simulink model "PLL_blocks"  (R2014a)
settings: Solver=ode45  StartTime=0.0  StopTime=10.0  RelTol=1e-3
libraries: simulink x12
settings Model: Creator=Tony  LastModifiedBy=Tony

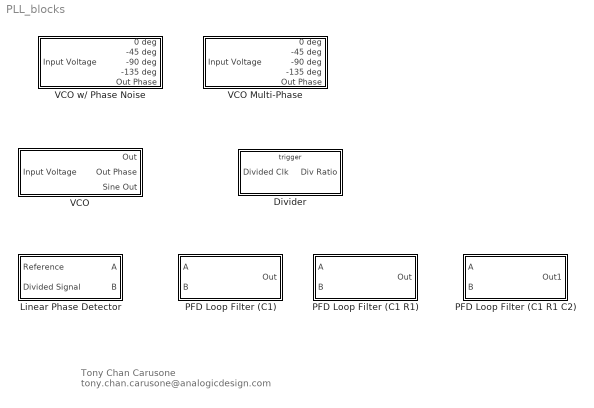
== system PLL_blocks ==
  note: Tony Chan Carusone
      | tony.chan.carusone@analogicdesign.com
  Divider : Subsystem
  Linear Phase Detector : Subsystem
  PFD Loop Filter (C1 R1 C2) : Subsystem  mask{Iu=25e-6, Id=25e-6, R1=6400, C1=16e-12, C2=1.6e-12}
      mask prompts: Iu "Loop Filter Pull Up Current (Iu)"; Id "Loop Filter Pull Down Current (Id)"
  PFD Loop Filter (C1 R1) : Subsystem  mask{Iu=25e-6, Id=25e-6, R1=8400, C1=16e-12}
      mask prompts: Iu "Loop Filter Pull Up Current (Iu)"; Id "Loop Filter Pull Down Current (Id)"
  PFD Loop Filter (C1) : Subsystem  mask{Iu=25e-6, Id=25e-6, C1=16e-12}
      mask prompts: Iu "Loop Filter Pull Up Current (Iu)"; Id "Loop Filter Pull Down Current (Id)"
  VCO : Subsystem  mask{Kvco=1e9*2*pi, Ac=1, fo=1000e6}
      mask prompts: fo "Default Frequency (fo)"
  VCO Multi-Phase : Subsystem  mask{Kvco=1e9*2*pi, fo=1000e6}
      mask prompts: fo "Default Frequency (fo)"
  VCO w/ Phase Noise : Subsystem  mask{Kvco=1e9*2*pi, fo=1000e6, h0=3e-15, N1=0}
      mask prompts: Kvco "Kvco [rad/s/V]"; fo "Nominal Frequency (fo) [Hz]"; h0 "White phase noise spectal density (rad^2/Hz)"; N1 "Low frequency phase noise (Hz^2*rad^2/Hz)"

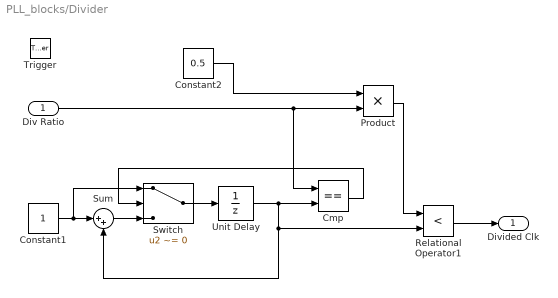
== system PLL_blocks/Divider ==
  Div Ratio : Inport
  Trigger : TriggerPort
  Cmp : RelationalOperator  Operator===  OutDataTypeStr=boolean
  Constant1 : Constant  OutDataTypeStr=int32
  Constant2 : Constant  Value=0.5
  Product : Product  RndMeth=Zero
  Relational Operator1 : RelationalOperator  Operator=<  OutDataTypeStr=boolean
  Sum : Sum  Inputs=|++
  Switch : Switch  Criteria=u2 ~= 0
  Unit Delay : UnitDelay  SampleTime=-1
  Divided Clk : Outport
  wires:
  Switch/1 -> Unit Delay/1
  Unit Delay/1 -> Sum/2, Relational Operator1/2, Cmp/2
  Relational Operator1/1 -> Divided Clk/1
  Product/1 -> Relational Operator1/1
  Constant2/1 -> Product/1
  Div Ratio/1 -> Product/2, Cmp/1
  Cmp/1 -> Switch/2
  Sum/1 -> Switch/3
  Constant1/1 -> Switch/1, Sum/1

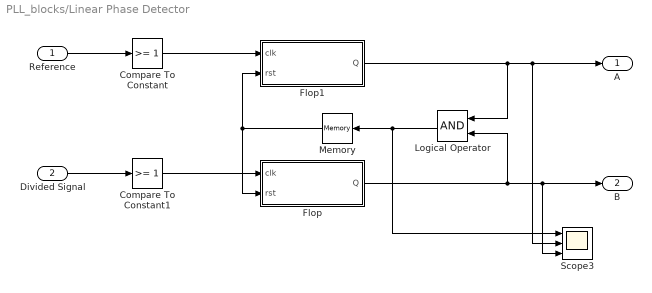
== system PLL_blocks/Linear Phase Detector ==
  Reference : Inport
  Divided Signal : Inport  Port=2
  Compare To Constant : simulink/Logic and Bit Operations/Compare To Constant  relop=>=  const=1  OutDataTypeStr=boolean  ZeroCross=off
  Compare To Constant1 : simulink/Logic and Bit Operations/Compare To Constant  relop=>=  const=1  OutDataTypeStr=boolean  ZeroCross=off
  Flop : Subsystem
  Flop1 : Subsystem
  Logical Operator : Logic  AllPortsSameDT=off  OutDataTypeStr=boolean
  Memory : Memory
  Scope3 : Scope  NumInputPorts=3
      settings: YMin=-1~-5~-5  YMax=2~5~5  SaveName=ScopeData4
  A : Outport
  B : Outport  Port=2
  wires:
  Memory/1 -> Flop1/2(rst), Flop/2(rst)
  Logical Operator/1 -> Memory/1, Scope3/1
  Compare To Constant1/1 -> Flop/1(clk)
  Divided Signal/1 -> Compare To Constant1/1
  Compare To Constant/1 -> Flop1/1(clk)
  Reference/1 -> Compare To Constant/1
  Flop/1(Q) -> Scope3/3, B/1, Logical Operator/2
  Flop1/1(Q) -> Scope3/2, A/1, Logical Operator/1

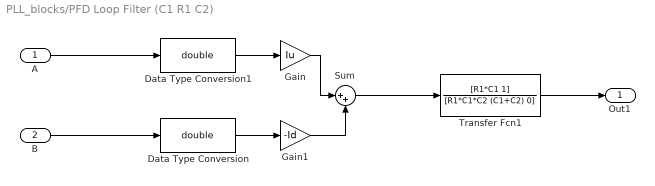
== system PLL_blocks/PFD Loop Filter (C1 R1 C2) ==
  A : Inport
  B : Inport  Port=2
  Data Type Conversion : DataTypeConversion  OutDataTypeStr=double
  Data Type Conversion1 : DataTypeConversion  OutDataTypeStr=double
  Gain : Gain  Gain=Iu
  Gain1 : Gain  Gain=-Id
  Sum : Sum  Inputs=|++
  Transfer Fcn1 : TransferFcn  Numerator=[R1*C1 1]  Denominator=[R1*C1*C2 (C1+C2) 0]
  Out1 : Outport
  wires:
  A/1 -> Data Type Conversion1/1
  B/1 -> Data Type Conversion/1
  Transfer Fcn1/1 -> Out1/1
  Sum/1 -> Transfer Fcn1/1
  Gain1/1 -> Sum/2
  Data Type Conversion/1 -> Gain1/1
  Gain/1 -> Sum/1
  Data Type Conversion1/1 -> Gain/1

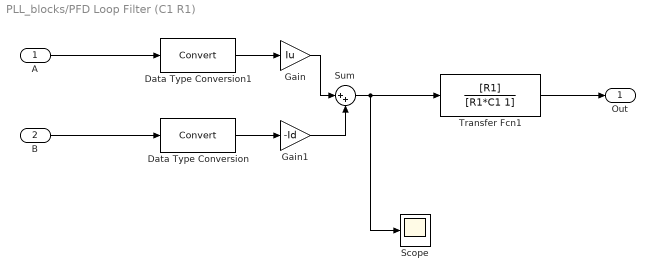
== system PLL_blocks/PFD Loop Filter (C1 R1) ==
  A : Inport
  B : Inport  Port=2
  Data Type Conversion : DataTypeConversion
  Data Type Conversion1 : DataTypeConversion
  Gain : Gain  Gain=Iu
  Gain1 : Gain  Gain=-Id
  Scope : Scope
      settings: YMin=-1  YMax=1  SaveName=ScopeData2
  Sum : Sum  Inputs=|++
  Transfer Fcn1 : TransferFcn  Numerator=[R1]  Denominator=[R1*C1 1]
  Out : Outport
  wires:
  A/1 -> Data Type Conversion1/1
  B/1 -> Data Type Conversion/1
  Transfer Fcn1/1 -> Out/1
  Sum/1 -> Transfer Fcn1/1, Scope/1
  Gain1/1 -> Sum/2
  Data Type Conversion/1 -> Gain1/1
  Gain/1 -> Sum/1
  Data Type Conversion1/1 -> Gain/1

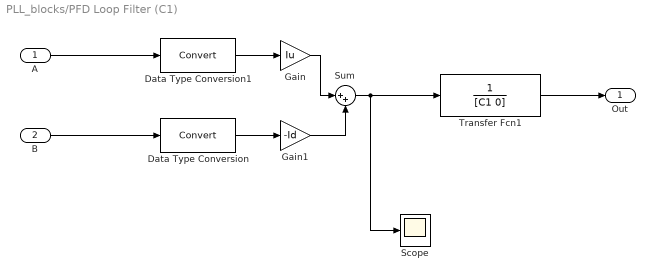
== system PLL_blocks/PFD Loop Filter (C1) ==
  A : Inport
  B : Inport  Port=2
  Data Type Conversion : DataTypeConversion
  Data Type Conversion1 : DataTypeConversion
  Gain : Gain  Gain=Iu
  Gain1 : Gain  Gain=-Id
  Scope : Scope
      settings: YMin=-1  YMax=1  SaveName=ScopeData2
  Sum : Sum  Inputs=|++
  Transfer Fcn1 : TransferFcn  Denominator=[C1 0]
  Out : Outport
  wires:
  A/1 -> Data Type Conversion1/1
  B/1 -> Data Type Conversion/1
  Transfer Fcn1/1 -> Out/1
  Sum/1 -> Transfer Fcn1/1, Scope/1
  Gain1/1 -> Sum/2
  Data Type Conversion/1 -> Gain1/1
  Gain/1 -> Sum/1
  Data Type Conversion1/1 -> Gain/1

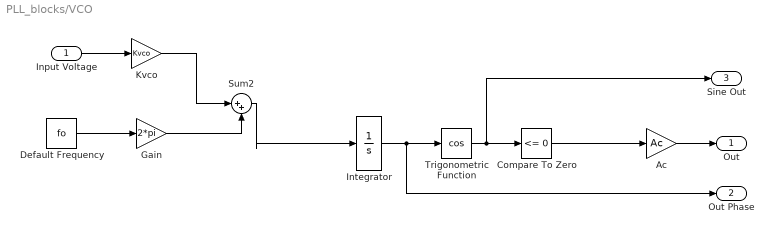
== system PLL_blocks/VCO ==
  Input Voltage : Inport
  Ac : Gain  Gain=Ac
  Compare To Zero : simulink/Logic and Bit Operations/Compare To Zero  relop=<=  OutDataTypeStr=uint8
  Default Frequency : Constant  Value=fo
  Gain : Gain  Gain=2*pi
  Integrator : Integrator
  Kvco : Gain  Gain=Kvco  OutDataTypeStr=Inherit: Inherit via back propagation
  Sum2 : Sum  Inputs=|++
  Trigonometric Function : Trigonometry  Operator=cos
  Out : Outport
  Out Phase : Outport  Port=2
  Sine Out : Outport  Port=3
  wires:
  Ac/1 -> Out/1
  Compare To Zero/1 -> Ac/1
  Trigonometric Function/1 -> Sine Out/1, Compare To Zero/1
  Default Frequency/1 -> Gain/1
  Input Voltage/1 -> Kvco/1
  Integrator/1 -> Out Phase/1, Trigonometric Function/1
  Sum2/1 -> Integrator/1
  Gain/1 -> Sum2/2
  Kvco/1 -> Sum2/1

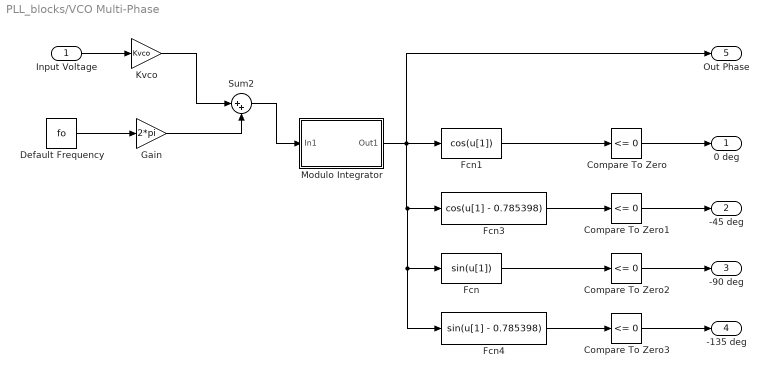
== system PLL_blocks/VCO Multi-Phase ==
  Input Voltage : Inport
  Compare To Zero{,1..3} (4 alike) : simulink/Logic and Bit Operations/Compare To Zero  relop=<=  OutDataTypeStr=uint8
  Default Frequency : Constant  Value=fo
  Fcn : Fcn
  Fcn1 : Fcn  Expr=cos(u[1])
  Fcn3 : Fcn  Expr=cos(u[1] - 0.785398)
  Fcn4 : Fcn  Expr=sin(u[1] - 0.785398)
  Gain : Gain  Gain=2*pi
  Kvco : Gain  Gain=Kvco  OutDataTypeStr=Inherit: Inherit via back propagation
  Modulo Integrator : Subsystem  AncestorBlock=comminteg2/Modulo Integrator/Modulo Integrator
  Sum2 : Sum  Inputs=|++
  0 deg : Outport
  -45 deg : Outport  Port=2
  -90 deg : Outport  Port=3
  -135 deg : Outport  Port=4
  Out Phase : Outport  Port=5
  wires:
  Compare To Zero3/1 -> -135 deg/1
  Compare To Zero2/1 -> -90 deg/1
  Compare To Zero1/1 -> -45 deg/1
  Compare To Zero/1 -> 0 deg/1
  Fcn/1 -> Compare To Zero2/1
  Fcn1/1 -> Compare To Zero/1
  Fcn3/1 -> Compare To Zero1/1
  Fcn4/1 -> Compare To Zero3/1
  Default Frequency/1 -> Gain/1
  Input Voltage/1 -> Kvco/1
  Modulo Integrator/1(Out1) -> Out Phase/1, Fcn1/1, Fcn3/1, Fcn/1, Fcn4/1
  Sum2/1 -> Modulo Integrator/1(In1)
  Gain/1 -> Sum2/2
  Kvco/1 -> Sum2/1

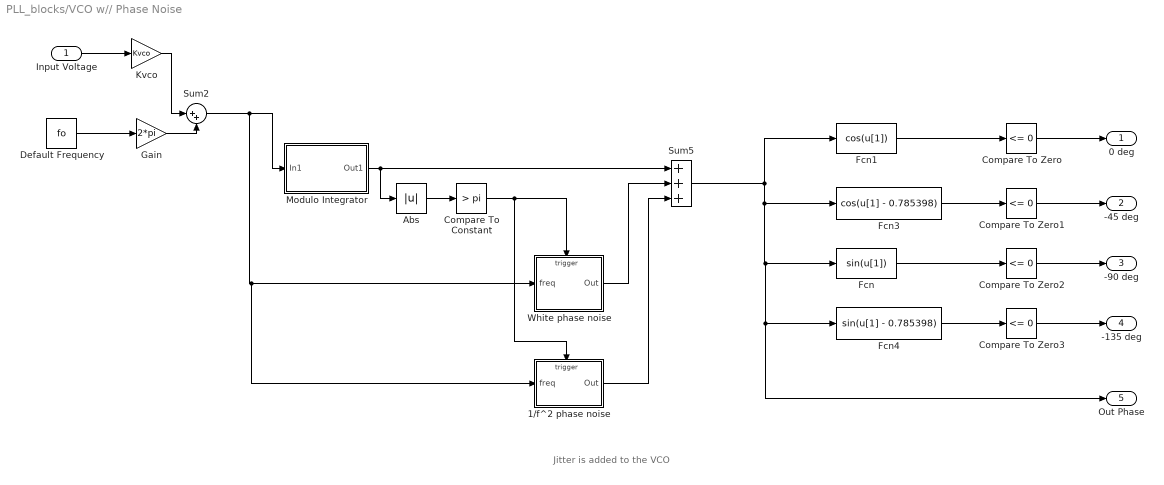
== system PLL_blocks/VCO w// Phase Noise ==
  note: Jitter is added to the VCO
  Input Voltage : Inport
  1/f^2 phase noise : Subsystem  TreatAsAtomicUnit=on
  Abs : Abs
  Compare To Constant : simulink/Logic and Bit Operations/Compare To Constant  relop=>  const=pi  OutDataTypeStr=boolean
  Compare To Zero{,1..3} (4 alike) : simulink/Logic and Bit Operations/Compare To Zero  relop=<=  OutDataTypeStr=uint8
  Default Frequency : Constant  Value=fo
  Fcn : Fcn
  Fcn1 : Fcn  Expr=cos(u[1])
  Fcn3 : Fcn  Expr=cos(u[1] - 0.785398)
  Fcn4 : Fcn  Expr=sin(u[1] - 0.785398)
  Gain : Gain  Gain=2*pi
  Kvco : Gain  Gain=Kvco  OutDataTypeStr=Inherit: Inherit via back propagation
  Modulo Integrator : Subsystem  AncestorBlock=comminteg2/Modulo Integrator/Modulo Integrator
  Sum2 : Sum  Inputs=|++
  Sum5 : Sum  Inputs=+++  SaturateOnIntegerOverflow=on  InputSameDT=on  OutDataTypeStr=Inherit: Same as first input
  White phase noise : Subsystem  TreatAsAtomicUnit=on
  0 deg : Outport
  -45 deg : Outport  Port=2
  -90 deg : Outport  Port=3
  -135 deg : Outport  Port=4
  Out Phase : Outport  Port=5
  wires:
  Compare To Constant/1 -> White phase noise/Trigger, 1/f^2 phase noise/Trigger
  Abs/1 -> Compare To Constant/1
  Sum5/1 -> Fcn1/1, Fcn3/1, Fcn/1, Out Phase/1, Fcn4/1
  1/f^2 phase noise/1(Out) -> Sum5/3
  White phase noise/1(Out) -> Sum5/2
  Sum2/1 -> Modulo Integrator/1(In1), White phase noise/1(freq), 1/f^2 phase noise/1(freq)
  Compare To Zero/1 -> 0 deg/1
  Modulo Integrator/1(Out1) -> Sum5/1, Abs/1
  Kvco/1 -> Sum2/1
  Gain/1 -> Sum2/2
  Input Voltage/1 -> Kvco/1
  Default Frequency/1 -> Gain/1
  Fcn4/1 -> Compare To Zero3/1
  Fcn3/1 -> Compare To Zero1/1
  Fcn1/1 -> Compare To Zero/1
  Fcn/1 -> Compare To Zero2/1
  Compare To Zero1/1 -> -45 deg/1
  Compare To Zero2/1 -> -90 deg/1
  Compare To Zero3/1 -> -135 deg/1

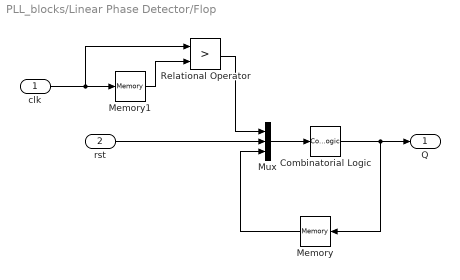
== system PLL_blocks/Linear Phase Detector/Flop ==
  clk : Inport
  rst : Inport  Port=2
  Combinatorial Logic : CombinatorialLogic  TruthTable=[0;1;0;0;1;1;0;0]
  Memory : Memory
  Memory1 : Memory
  Mux : Mux  Inputs=3
  Relational Operator : RelationalOperator  Operator=>  OutDataTypeStr=boolean
  Q : Outport
  wires:
  Relational Operator/1 -> Mux/1
  Memory1/1 -> Relational Operator/2
  clk/1 -> Memory1/1, Relational Operator/1
  Memory/1 -> Mux/3
  Combinatorial Logic/1 -> Q/1, Memory/1
  rst/1 -> Mux/2
  Mux/1 -> Combinatorial Logic/1

== system PLL_blocks/Linear Phase Detector/Flop1 ==
  clk : Inport
  rst : Inport  Port=2
  Combinatorial Logic : CombinatorialLogic  TruthTable=[0;1;0;0;1;1;0;0]
  Memory : Memory
  Memory1 : Memory
  Mux : Mux  Inputs=3
  Relational Operator : RelationalOperator  Operator=>  OutDataTypeStr=boolean
  Q : Outport
  wires:
  Relational Operator/1 -> Mux/1
  Memory1/1 -> Relational Operator/2
  clk/1 -> Memory1/1, Relational Operator/1
  Memory/1 -> Mux/3
  Combinatorial Logic/1 -> Memory/1, Q/1
  rst/1 -> Mux/2
  Mux/1 -> Combinatorial Logic/1

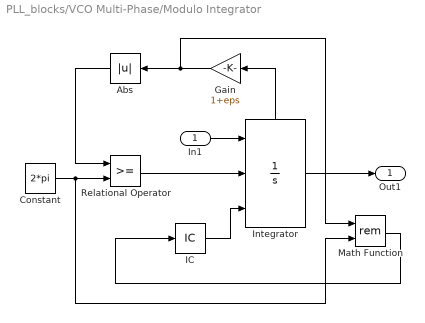
== system PLL_blocks/VCO Multi-Phase/Modulo Integrator ==
  In1 : Inport
  Abs : Abs  SaturateOnIntegerOverflow=on
  Constant : Constant  Value=2*pi
  Gain : Gain  Gain=1+eps  SaturateOnIntegerOverflow=on  OutDataTypeStr=Inherit: Same as input  ParamDataTypeStr=Inherit: Same as input
  IC : InitialCondition  Value=0
  Integrator : Integrator  ExternalReset=rising  InitialConditionSource=external  UpperSaturationLimit=1  LowerSaturationLimit=0  ShowStatePort=on
  Math Function : Math  Operator=rem  SaturateOnIntegerOverflow=on
  Relational Operator : RelationalOperator  InputSameDT=on
  Out1 : Outport
  wires:
  Gain/1 -> Math Function/1, Abs/1
  Integrator/State -> Gain/1
  Constant/1 -> Relational Operator/2, Math Function/2
  Relational Operator/1 -> Integrator/2
  Abs/1 -> Relational Operator/1
  Math Function/1 -> IC/1
  Integrator/1 -> Out1/1
  In1/1 -> Integrator/1
  IC/1 -> Integrator/3

== system PLL_blocks/VCO w// Phase Noise/1//f^2 phase noise ==
  note: Filter rolls off at -20dB/dec
      | with gain of
      | (freq/1 [Hz]) at 1 Hz
  note: This point is white noise with a variance of
      | N1 [rad^2*Hz] / freq [Hz]
  freq : Inport  LatchByDelayingOutsideSignal=on
  Trigger : TriggerPort
  1st-Order Filter : DiscreteFilter  Numerator=2*pi  Denominator=[1 -1]
  Fcn : Fcn  Expr=1/sqrt(u)
  Product : Product  SaturateOnIntegerOverflow=on  InputSameDT=on  OutDataTypeStr=Inherit: Same as first input
  Random Number : RandomNumber  Variance=N1/2  Seed=4987
  Out : Outport  InitialOutput=0
  wires:
  freq/1 -> Fcn/1
  1st-Order Filter/1 -> Out/1
  Random Number/1 -> Product/1
  Product/1 -> 1st-Order Filter/1
  Fcn/1 -> Product/2

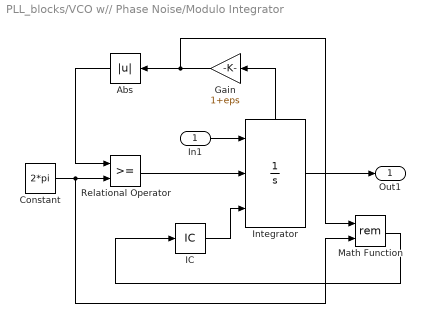
== system PLL_blocks/VCO w// Phase Noise/Modulo Integrator ==
  In1 : Inport
  Abs : Abs  SaturateOnIntegerOverflow=on
  Constant : Constant  Value=2*pi
  Gain : Gain  Gain=1+eps  SaturateOnIntegerOverflow=on  OutDataTypeStr=Inherit: Same as input  ParamDataTypeStr=Inherit: Same as input
  IC : InitialCondition  Value=0
  Integrator : Integrator  ExternalReset=rising  InitialConditionSource=external  UpperSaturationLimit=1  LowerSaturationLimit=0  ShowStatePort=on
  Math Function : Math  Operator=rem  SaturateOnIntegerOverflow=on
  Relational Operator : RelationalOperator  InputSameDT=on
  Out1 : Outport
  wires:
  IC/1 -> Integrator/3
  In1/1 -> Integrator/1
  Integrator/1 -> Out1/1
  Math Function/1 -> IC/1
  Abs/1 -> Relational Operator/1
  Relational Operator/1 -> Integrator/2
  Constant/1 -> Math Function/2, Relational Operator/2
  Integrator/State -> Gain/1
  Gain/1 -> Abs/1, Math Function/1

== system PLL_blocks/VCO w// Phase Noise/White phase noise ==
  note: Variance should be h0 [rad^2/Hz] * freq [Hz]
  freq : Inport  LatchByDelayingOutsideSignal=on
  Trigger : TriggerPort
  Fcn : Fcn  Expr=sqrt(u)
  Product : Product  SaturateOnIntegerOverflow=on  InputSameDT=on  OutDataTypeStr=Inherit: Same as first input
  Random Number : RandomNumber  Variance=h0/2  Seed=1238
  Out : Outport  InitialOutput=0
  wires:
  freq/1 -> Fcn/1
  Fcn/1 -> Product/2
  Product/1 -> Out/1
  Random Number/1 -> Product/1
